simulink model "ddpg_new_try1_sim_quad_delay"  (R2021a)
settings: Solver=VariableStepAuto  StartTime=0.0  StopTime=10.0  RelTol=1e-3
values from neighbouring files (symbols this model uses):
  Ts = 0.01    [A2C_2b_new_try1_quad.m]    (also in A2C_3ob_try1_quad.m; A2C_new_try1_quad.m; A2c_2ob_new_try2_Conactor.m; DQN_new_try1_quad.m)
undefined symbols (not defined in the file or in its folder): DiscIntNeverNeededParam
libraries: simulink x2, rllib x1
settings Model: Creator=SHRENI MALYALA  LastModifiedBy=SHRENI MALYALA

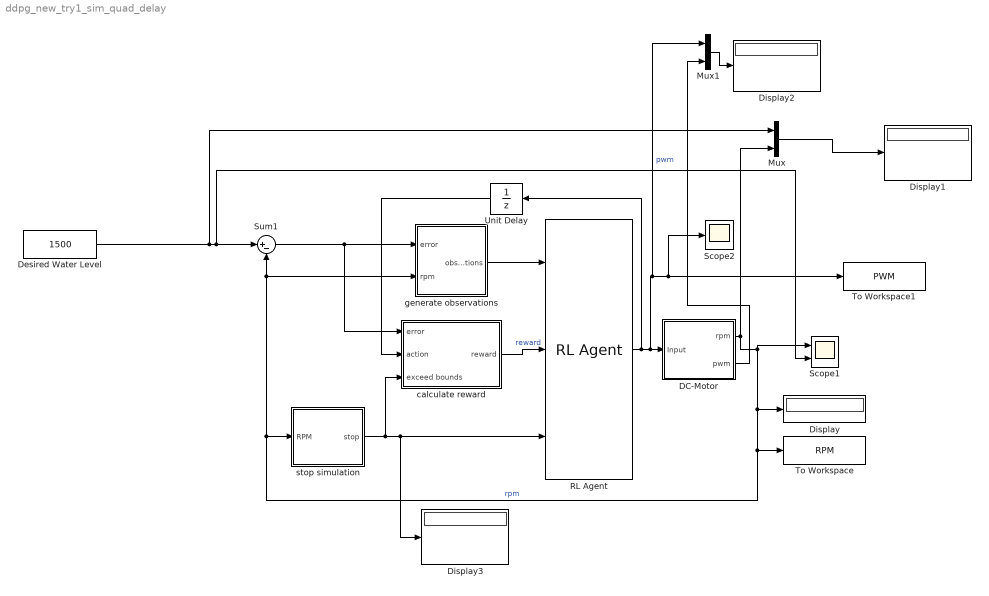
== system ddpg_new_try1_sim_quad_delay ==
  DC-Motor : Subsystem
  Desired Water Level : Constant  Value=1500
  Display{,1..3} (4 alike) : Display
  Mux : Mux  Inputs=2
  Mux1 : Mux  Inputs=2
  RL Agent : rllib/RL Agent  Agent=agent  ExternalActionAsInput=off  ProvideCumRwd=off  TreatAsDirectFeedthrough=on
  Scope1 : Scope  NumInputPorts=2
  Scope2 : Scope
  Sum1 : Sum  Inputs=|+-  SaturateOnIntegerOverflow=on
  To Workspace : ToWorkspace  VariableName=RPM  SampleTime=-1
  To Workspace1 : ToWorkspace  VariableName=PWM  SaveFormat=Timeseries  SampleTime=-1
  Unit Delay : UnitDelay  SampleTime=-1  HasFrameUpgradeWarning=on
  calculate reward : Subsystem
  generate observations : Subsystem
  stop simulation : Subsystem
  wires:
  Mux/1 -> Display1/1
  generate observations/1(observations) -> RL Agent/1
  Sum1/1 -> calculate reward/1(error), generate observations/1(error)
  calculate reward/1(reward) -> RL Agent/2  "reward"
  DC-Motor/1(rpm) -> Scope1/1, stop simulation/1(RPM), generate observations/2(rpm), Sum1/2, To Workspace/1, Display/1, Mux/2  "rpm"
  stop simulation/1(stop) -> Display3/1, RL Agent/3, calculate reward/3(exceed bounds)
  Desired Water Level/1 -> Scope1/2, Sum1/1, Mux/1
  RL Agent/1 -> Unit Delay/1, Mux1/1, Scope2/1, To Workspace1/1, DC-Motor/1(Input)  "pwm"
  DC-Motor/2(pwm) -> Mux1/2
  Unit Delay/1 -> calculate reward/2(action)
  Mux1/1 -> Display2/1

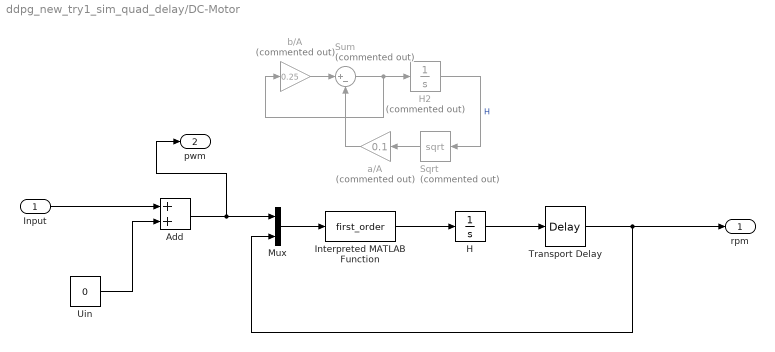
== system ddpg_new_try1_sim_quad_delay/DC-Motor ==
  Input : Inport
  Add : Sum
  H : Integrator  InitialCondition=3  LimitOutput=on  LowerSaturationLimit=0
  H2 : Integrator  Commented=on  InitialCondition=3  LimitOutput=on  LowerSaturationLimit=0
  Interpreted MATLAB Function : MATLABFcn  MATLABFcn=first_order  OutputDimensions=1
  Mux : Mux  Inputs=2
  Sqrt : Sqrt  Commented=on  OutputSignalType=real  SaturateOnIntegerOverflow=on
  Sum : Sum  Commented=on  Inputs=|+-  SaturateOnIntegerOverflow=on
  Transport Delay : TransportDelay  DelayTime=0.03
  Uin : Constant  Value=0
  a/A : Gain  Commented=on  Gain=0.1  SaturateOnIntegerOverflow=on  OutDataTypeStr=Inherit: Same as input  ParamDataTypeStr=Inherit: Same as input
  b/A : Gain  Commented=on  Gain=0.25  SaturateOnIntegerOverflow=on  OutDataTypeStr=Inherit: Same as input  ParamDataTypeStr=Inherit: Same as input
  rpm : Outport  VectorParamsAs1DForOutWhenUnconnected=off
  pwm : Outport  Port=2  VectorParamsAs1DForOutWhenUnconnected=off
  wires:
  b/A/1 -> Sum/1
  Sum/1 -> b/A/1, H2/1
  H2/1 -> Sqrt/1  "H"
  Sqrt/1 -> a/A/1
  a/A/1 -> Sum/2
  Mux/1 -> Interpreted MATLAB Function/1
  Interpreted MATLAB Function/1 -> H/1
  H/1 -> Transport Delay/1
  Input/1 -> Add/1
  Uin/1 -> Add/2
  Add/1 -> pwm/1, Mux/1
  Transport Delay/1 -> rpm/1, Mux/2

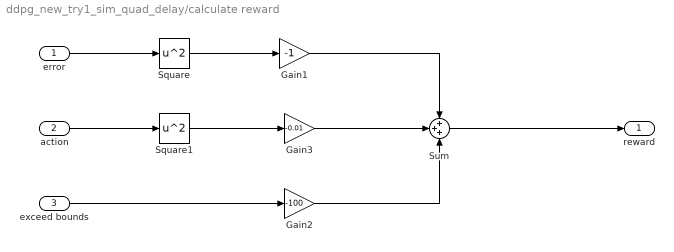
== system ddpg_new_try1_sim_quad_delay/calculate reward ==
  error : Inport
  action : Inport  Port=2
  exceed bounds : Inport  Port=3
  Gain1 : Gain  Gain=-1
  Gain2 : Gain  Gain=-100
  Gain3 : Gain  Gain=-0.01
  Square : Math  Operator=square  SaturateOnIntegerOverflow=on
  Square1 : Math  Operator=square  SaturateOnIntegerOverflow=on
  Sum : Sum  Inputs=+++  OutDataTypeStr=double
  reward : Outport  VectorParamsAs1DForOutWhenUnconnected=off
  wires:
  Sum/1 -> reward/1
  exceed bounds/1 -> Gain2/1
  action/1 -> Square1/1
  error/1 -> Square/1
  Square1/1 -> Gain3/1
  Square/1 -> Gain1/1
  Gain1/1 -> Sum/1
  Gain3/1 -> Sum/2
  Gain2/1 -> Sum/3

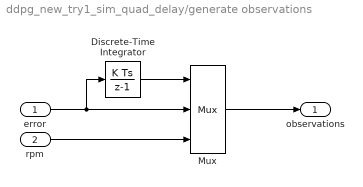
== system ddpg_new_try1_sim_quad_delay/generate observations ==
  error : Inport
  rpm : Inport  Port=2
  Discrete-Time Integrator : DiscreteIntegrator  SampleTime=Ts  ICPrevOutput=DiscIntNeverNeededParam  ICPrevScaledInput=DiscIntNeverNeededParam
  Mux : Mux  Inputs=3
  observations : Outport  VectorParamsAs1DForOutWhenUnconnected=off
  wires:
  rpm/1 -> Mux/3
  Discrete-Time Integrator/1 -> Mux/1
  error/1 -> Discrete-Time Integrator/1, Mux/2
  Mux/1 -> observations/1

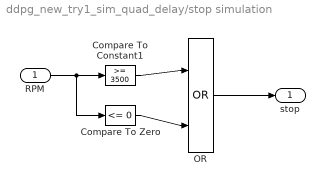
== system ddpg_new_try1_sim_quad_delay/stop simulation ==
  RPM : Inport
  Compare To Constant1 : simulink/Logic and Bit Operations/Compare To Constant  relop=>=  const=3500  OutDataTypeStr=boolean
  Compare To Zero : simulink/Logic and Bit Operations/Compare To Zero  relop=<=  OutDataTypeStr=boolean
  OR : Logic  Operator=OR  IconShape=distinctive  AllPortsSameDT=off  OutDataTypeStr=boolean
  stop : Outport  VectorParamsAs1DForOutWhenUnconnected=off
  wires:
  RPM/1 -> Compare To Zero/1, Compare To Constant1/1
  Compare To Zero/1 -> OR/2
  Compare To Constant1/1 -> OR/1
  OR/1 -> stop/1
